simulink model "Lagaya_RJ_MATLAB_No3"  (R2024a)
settings: Solver=VariableStepAuto  StartTime=0.0  StopTime=10.0  RelTol=1e-3
settings Model: Creator=Rod Joshua Lagaya  LastModifiedBy=Rod Joshua Lagaya

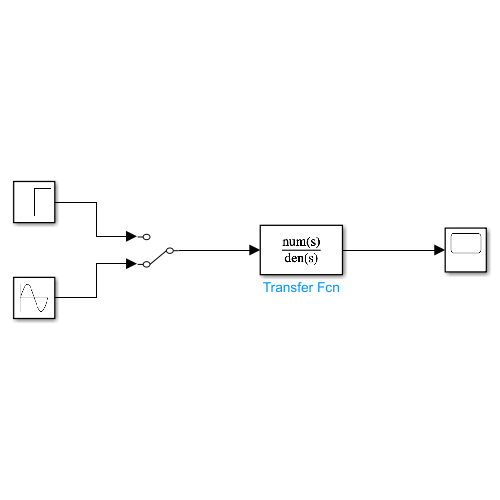
[thumbnail: Simulink's stored preview of the top-level diagram]
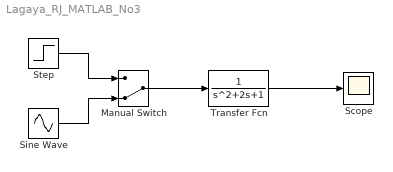
== system Lagaya_RJ_MATLAB_No3 ==
  Manual Switch : ManualSwitch  CurrentSetting=0
  Scope : Scope
  Sine Wave : Sin  SampleTime=0
  Step : Step  Time=0  SampleTime=0
  Transfer Fcn : TransferFcn
  wires:
  Manual Switch/1 -> Transfer Fcn/1
  Step/1 -> Manual Switch/1
  Transfer Fcn/1 -> Scope/1
  Sine Wave/1 -> Manual Switch/2
